simulink model "Conversor_BUCK"  (R2025a)
settings: Solver=VariableStepAuto  StartTime=0.0  StopTime=10.0  RelTol=1e-3
settings Model: Creator=Ruth Juana  LastModifiedBy=Ruth Juana

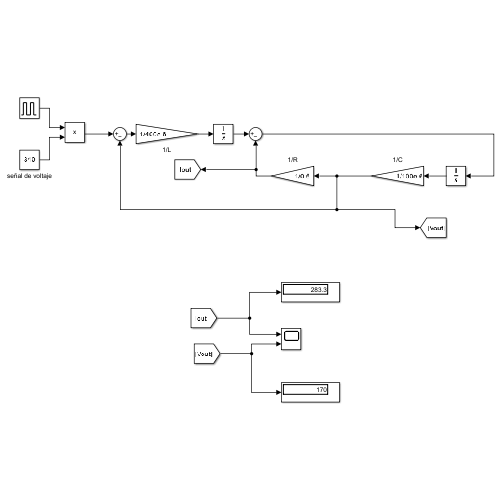
[thumbnail: Simulink's stored preview of the top-level diagram]
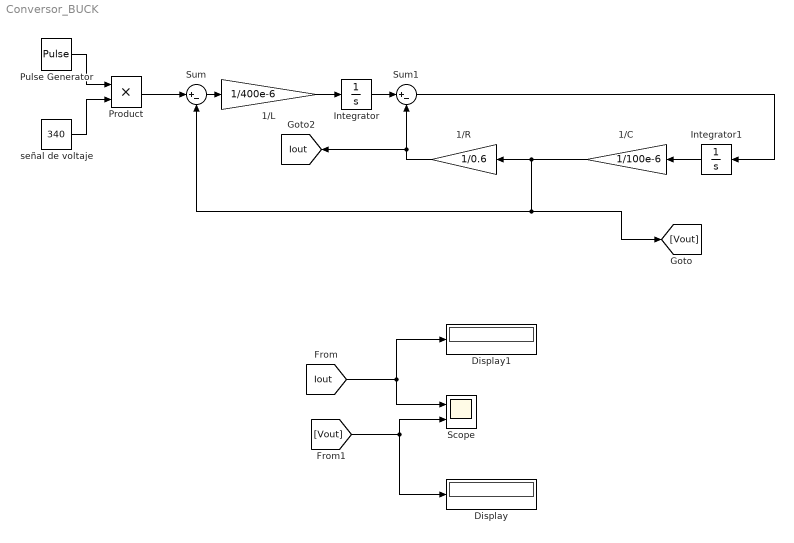
== system Conversor_BUCK ==
  1/C : Gain  Gain=1/100e-6
  1/L : Gain  Gain=1/400e-6
  1/R : Gain  Gain=1/0.6
  Display : Display
  Display1 : Display
  Integrator : Integrator
  Integrator1 : Integrator
  Product : Product
  Pulse Generator : DiscretePulseGenerator  PulseType=Time based  Period=1/20e3  PulseWidth=0.5*100
  Scope : Scope  NumInputPorts=2
      settings: ActiveDisplayYMinimum=-191.12110162531121  ActiveDisplayYMaximum=400.9173822300337
  Sum : Sum  Inputs=|+-
  Sum1 : Sum  Inputs=|+-
  señal de voltaje : Constant  Value=340
  tag scope: Iout=global
  wires:
  señal de voltaje/1 -> Product/2
  Pulse Generator/1 -> Product/1
  Product/1 -> Sum/1
  Sum/1 -> 1/L/1
  1/L/1 -> Integrator/1
  Integrator/1 -> Sum1/1
  Sum1/1 -> Integrator1/1
  1/C/1 -> 1/R/1, Sum/2, [Vout]
  1/R/1 -> Sum1/2, [Iout]
  Integrator1/1 -> 1/C/1
  [Iout] -> Display1/1, Scope/1
  [Vout] -> Display/1, Scope/2
